simulink model "s_servo_pos_cntrl"  (R2018b)
settings: Solver=ode4  StartTime=0.0  StopTime=5  FixedStep=0.002  RelTol=1e-3  AbsTol=1e-6  EnableMultiTasking=on
values from neighbouring files (symbols this model uses):
  K = 10    [setup_servo_pos_cntrl.m]
  kd = 0    [setup_servo_pos_cntrl.m]
  ki = 0    [setup_servo_pos_cntrl.m]
  kp = 0    [setup_servo_pos_cntrl.m]
  tau = 0.1    [setup_servo_pos_cntrl.m]
undefined symbols (not defined in the file or in its folder): VMAX_DAC
libraries: quarc_library x1
settings Model: ExtModeTrigDuration=10000  Creator=MLevis  LastModifiedBy=MLevis
settings SolverCC: AutoScaleAbsTol=off  PositivePriorityOrder=on
settings DataIOCC: SaveFormat=Array  SignalLoggingSaveFormat=ModelDataLogs
settings OptimizationCC: BlockReduction=off  BooleanDataType=off  OptimizeBlockIOStorage=off  BufferReuse=off  GlobalBufferReuse=off  ExpressionFolding=off  ExpressionDepthLimit=2147483647  LocalBlockOutputs=off  InitFltsAndDblsToZero=on  LifeSpan=inf  OptimizeDataStoreBuffers=off  BusAssignmentInplaceUpdate=off
settings DebuggingCC: SaveWithParameterizedLinksMsg=none  UnderspecifiedInitializationDetection=Classic  MergeDetectMultiDrivingBlocksExec=none  SignalResolutionControl=TryResolveAllWithWarning  MultiTaskDSMMsg=warning  MultiTaskCondExecSysMsg=none  FcnCallInpInsideContextMsg=warning  StateNameClashWarn=warning  SFUnexpectedBacktrackingDiag=warning  SFNoUnconditionalDefaultTransitionDiag=warning  SFExecutionAtInitializationDiag=none
settings HardwareCC: ProdBitPerPointer=32  ProdBitPerSizeT=32  ProdBitPerPtrDiffT=32  ProdLargestAtomicFloat=None  ProdIntDivRoundTo=Undefined  ProdEndianess=Unspecified  ProdWordSize=32  ProdHWDeviceType=32-bit Generic  TargetHWDeviceType=32-bit Generic
settings ModelReferenceCC: PropagateSignalLabelsOutOfModel=off
settings RTWCC: SystemTargetFile=quarc_windows.tlc  TemplateMakefile=quarc_default_tmf  Description=Quarc Win32 Target
settings CodeAppCC: StateflowObjectComments=on
settings STFCustomTargetCC: TargetFcnLib=ansi_tfl_tmw.mat  TargetPreCompLibLocation=C:\PROGRA~3\QUARC\lib\2018b\windows\release  CPPClassGenCompliant=on  GRTInterface=on  SystemTargetFile=quarc_windows.tlc
settings GRTTargetCC: TargetFcnLib=ansi_tfl_tmw.mat  TargetPreCompLibLocation=C:\PROGRA~3\QUARC\lib\2018b\windows\release  TargetLangStandard=C89/C90 (ANSI)  ParMdlRefBuildCompliant=off  CompOptLevelCompliant=off  ConcurrentExecutionCompliant=off  CombineOutputUpdateFcns=off  MatFileLogging=off  GRTInterface=on  UseToolchainInfoCompliant=off  ExtMode=on  ExtModeMexFile=quarc_comm
settings ConfigComp: CovMetricSettings=dw  CovHtmlReporting=on  CovSaveCumulativeToWorkspaceVar=on  CovSaveSingleToWorkspaceVar=on

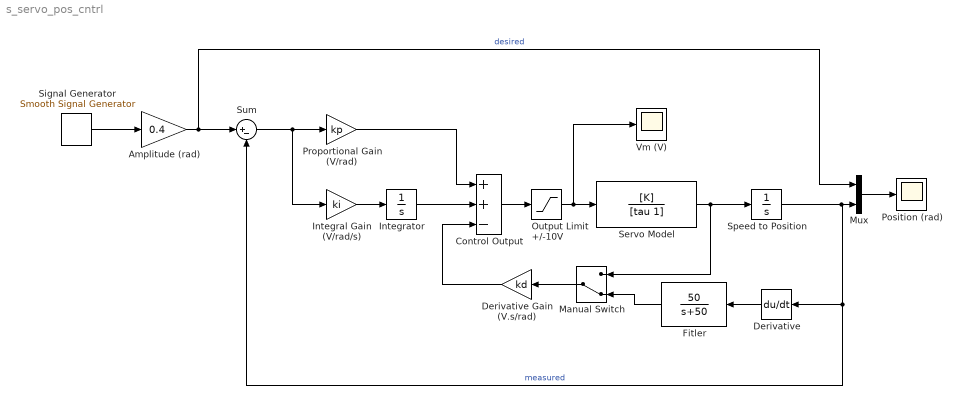
== system s_servo_pos_cntrl ==
  Amplitude (rad) : Gain  Gain=0.4  SaturateOnIntegerOverflow=on  OutDataTypeStr=Inherit: Same as input  ParamDataTypeStr=Inherit: Same as input
  Control Output : Sum  Inputs=++-
  Derivative : Derivative
  Derivative Gain (V.s/rad) : Gain  Gain=kd
  Fitler : TransferFcn  Numerator=[50]  Denominator=[1 50]
  Integral Gain (V/rad/s) : Gain  Gain=ki
  Integrator : Integrator  UpperSaturationLimit=VMAX_DAC  LowerSaturationLimit=-VMAX_DAC
  Manual Switch : ManualSwitch  CurrentSetting=0
  Mux : Mux  Inputs=2
  Output Limit +/-10V : Saturate  UpperLimit=10  LowerLimit=-10
  Position (rad) : Scope
  Proportional Gain (V/rad) : Gain  Gain=kp
  Servo Model : TransferFcn  Numerator=[K]  Denominator=[tau 1]
  Signal Generator : quarc_library/Sources/Signals/Smooth Signal Generator  signal_type=Square  source=Internal (dialog parameters)  amplitude=1  frequency=0.4  initial_phase=0  sample_time=qc_get_step_size  output_cos=off
      settings: SourceProductName=QUARC Targets
  Speed to Position : Integrator
  Sum : Sum  Inputs=|+-
  Vm (V) : Scope
  wires:
  Mux/1 -> Position (rad)/1
  Signal Generator/1 -> Amplitude (rad)/1
  Servo Model/1 -> Manual Switch/1, Speed to Position/1
  Amplitude (rad)/1 -> Sum/1, Mux/1  "desired"
  Proportional Gain (V/rad)/1 -> Control Output/1
  Control Output/1 -> Output Limit +/-10V/1
  Integral Gain (V/rad/s)/1 -> Integrator/1
  Derivative Gain (V.s/rad)/1 -> Control Output/3
  Integrator/1 -> Control Output/2
  Sum/1 -> Integral Gain (V/rad/s)/1, Proportional Gain (V/rad)/1
  Output Limit +/-10V/1 -> Vm (V)/1, Servo Model/1
  Speed to Position/1 -> Derivative/1, Sum/2, Mux/2  "measured"
  Manual Switch/1 -> Derivative Gain (V.s/rad)/1
  Fitler/1 -> Manual Switch/2
  Derivative/1 -> Fitler/1
